simulink model "mech_ballistic_kin_fric"  (Simulink 6.0)
settings: Solver=ode45  StartTime=0.0  StopTime=inf  RelTol=1e-3
values from neighbouring files (symbols this model uses):
  m = 161    [mech_transmission_data.mat]
  N = 270    [mech_transmission_data.mat]
libraries: mblibv1 x10, simulink x1
settings Model: Creator=dkennedy  LastModifiedBy=batserve  ExtModeAutoUpdateStatusClock=off
settings DataIOCC: SignalLoggingName=sigsOut
settings DebuggingCC: CheckExecutionContextPreStartOutputMsg=on  CheckExecutionContextRuntimeOutputMsg=on  SolverPrmCheckMsg=none
settings HardwareCC: TargetUnknown=on

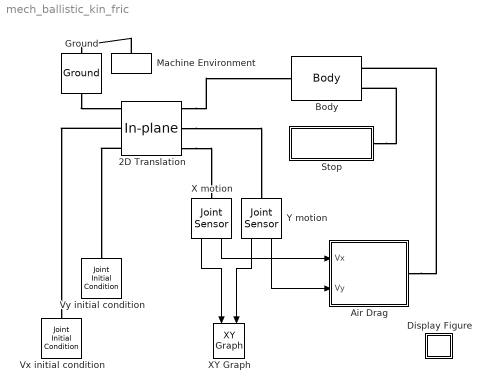
== system mech_ballistic_kin_fric ==
  2D Translation : mblibv1/Joints/In-plane  PhysicalDomain=mechanical  SubClassName=Unknown  LeftPortType=blob  RightPortType=blob  LConnTagsString=__newl0|SA1|SA2  RConnTagsString=__newr0|SA1|SA2  NumSAPorts=4  CutJoint=off  MarkAsCut=off  Primitives=prismatic_prismatic  PrimitiveProps=P1$WORLD$[1 0 0]$prismatic#P2$WORLD$[0 1 0]$prismatic  DialogClass=JointBlock
  Air Drag : Subsystem  mask(Air friction model){Cd=0}
      mask prompts: Cd "Drag Coefficient"
      mask help: Models aerodynamic drag. The drag coefficient Cd is a mask block parameter. Cd = 0 corresponds to zero drag. Cd = 2 corresponds to a sphere.
      mask init:
      | 0;
      mask Help: Enter aerodynamic drag coefficient Cd.  The block generates a three-vector of air friction as a function of 2D input velocity.
  Body : mblibv1/Bodies/Body  PhysicalDomain=mechanical  SubClassName=Unknown  LeftPortType=workingframe  RightPortType=workingframe  LConnTagsString=CS1  RConnTagsString=CS2|CG  DialogClass=MechanicalBodyBlock  Mass=100  MassUnits=kg  InertiaUnits=kg*m^2  Inertia=eye(3)*10  Shape=Cylinder  ShapeDims=[1 1]  ShapeUnits=m  ShapeUse=false  Density=1  DensityUnits=kg/m^3  DensityUse=false  CG=Right$CG$[0 0 0]$WORLD$WORLD$m$[0 0 0]$Euler X-Y-Z$deg$WORLD$true  WorkingFrames=Left$CS1$[0 0 0]$WORLD$CG$m$[0 0 0]$Euler X-Y-Z$deg$WORLD$true#Right$CS2$[0 0 0]$WORLD$CG$m$[0 0 0]$Euler X-Y-Z$deg$WORLD$true
  Display Figure : Subsystem  Tag=Help  Description="Help callback for ballistic kinetic friction model: mech_ballistic_kin_fric.  Opens Help browser to Type 19 marker at documentation for this tutorial model."
      settings: OpenFcn=pmhelpview([docroot '/toolbox/physmod/mech/mech.map'], 'mech_ballistic_kin_fric_help');
      mask Type: Help callback
      mask Display: image(imread('info.bmp'))
  Ground : mblibv1/Bodies/Ground  Orientation=down  Opaque=on  LeftPortType=env  RightPortType=workingframe  PhysicalDomain=Mechanical  DialogClass=GroundBlock  CoordPosition=[0 0 0]  CoordPositionUnits=m  StateVectorMgrId=-1  MachineId=[0 0]  ShowEnvPort=on
  Machine Environment : mblibv1/Bodies/Machine Environment  Tag=Factory ground  Orientation=up  DialogController=MECH.DialogSource  Opaque=on  PortType=env  PhysicalDomain=Mechanical  DialogTemplateClass=MECH.MachineEnvironment  SyncWhenCopied=off  Gravity=[0 -9.81 0]  GravityUnits=m/s^2  GravityAsSignal=off  Dimensionality=3D Only  AnalysisType=Forward dynamics  LinearAssemblyTolerance=1e-3  LinearAssemblyToleranceUnits=m  AngularAssemblyTolerance=1e-3  AngularAssemblyToleranceUnits=rad  ConstraintSolverType=Stabilizing  ConstraintRelTolerance=1e-4  ConstraintAbsTolerance=1e-4  UseRobustSingularityHandling=off  StatePerturbationType=Fixed  PerturbationSize=1e-5  VisualizeMachine=on
  Stop : Subsystem  Orientation=left
  Vx initial condition : mblibv1/Sensors &  Actuators/Joint Initial Condition  Orientation=up  Opaque=on  PhysicalDomain=Mechanical  DialogClass=InitialConditionBlock  Primitive=P1  CoordPosition=0.0  Velocity=98.0  AngleUnits=deg  ArcVelocityUnits=deg/s  CoordPositionUnits=m  VelocityUnits=m/s  InitialConditions=P1$true$0.0$m$deg$98.0$m/s$deg/s#P2$false$0$m$rad$0$m/s$rad/s#P3$false$0$m$rad$0$m/s$rad/s#R1$false$0$m$rad$0$m/s$rad/s#R2$false$0$m$rad$0$m/s$rad/s#R3$false$0$m$rad$0$m/s$rad/s#S$false$0$m$rad$0$m/s$rad/s
  Vy initial condition : mblibv1/Sensors &  Actuators/Joint Initial Condition  Orientation=up  Opaque=on  PhysicalDomain=Mechanical  DialogClass=InitialConditionBlock  Primitive=P2  CoordPosition=0.0  Velocity=69.0  AngleUnits=deg  ArcVelocityUnits=deg/s  CoordPositionUnits=m  VelocityUnits=m/s  InitialConditions=P1$false$0$m$rad$0$m/s$rad/s#P2$true$0.0$m$deg$69.0$m/s$deg/s#P3$false$0$m$rad$0$m/s$rad/s#R1$false$0$m$rad$0$m/s$rad/s#R2$false$0$m$rad$0$m/s$rad/s#R3$false$0$m$rad$0$m/s$rad/s#S$false$0$m$rad$0$m/s$rad/s
  X motion : mblibv1/Sensors &  Actuators/Joint Sensor  Orientation=down  Opaque=on  PhysicalDomain=Mechanical  PortType=blob  Muxed=off  Pose=off  Angle=on  AngleUnits=deg  ArcVelocity=off  ArcVelocityUnits=deg/s  ArcAcceleration=off  ArcAccelerationUnits=deg/s^2  CoordPosition=on  CoordPositionUnits=m  Velocity=on  VelocityUnits=m/s  Acceleration=off  AccelerationUnits=m/s^2  Quaternion=on  QuaternionDT=off  QuaternionDDT=off  QuaternionUnits=off  OutputVector=[ 1 1 ]  ActiveIO=on  Width=2  DialogClass=MechanicalSensorBlock  Primitive=P1  Force=off  ForceUnits=N  Torque=off  TorqueUnits=N-m  ReferenceFrame=Absolute (INERTIAL)  ReactionSensedSide=Base  ReactionReferenceFrame=Absolute (World)  ReactionForce=off  ReactionForceUnits=N  ReactionMoment=off  ReactionMomentUnits=N-m
  XY Graph : simulink/Sinks/XY Graph  Orientation=down  xmin=0  xmax=1500  ymin=0  ymax=400  st=-1
  Y motion : mblibv1/Sensors &  Actuators/Joint Sensor  Orientation=down  Opaque=on  PhysicalDomain=Mechanical  PortType=blob  Muxed=off  Pose=off  Angle=on  AngleUnits=deg  ArcVelocity=off  ArcVelocityUnits=deg/s  ArcAcceleration=off  ArcAccelerationUnits=deg/s^2  CoordPosition=on  CoordPositionUnits=m  Velocity=on  VelocityUnits=m/s  Acceleration=off  AccelerationUnits=m/s^2  Quaternion=on  QuaternionDT=off  QuaternionDDT=off  QuaternionUnits=off  OutputVector=[ 1 1 ]  ActiveIO=on  Width=2  DialogClass=MechanicalSensorBlock  Primitive=P2  Force=off  ForceUnits=N  Torque=off  TorqueUnits=N-m  ReferenceFrame=Absolute (INERTIAL)  ReactionSensedSide=Base  ReactionReferenceFrame=Absolute (World)  ReactionForce=off  ReactionForceUnits=N  ReactionMoment=off  ReactionMomentUnits=N-m
  wires:
  X motion/2 -> Air Drag/1(Vx)
  Y motion/2 -> Air Drag/2(Vy)
  X motion/1 -> XY Graph/1
  Y motion/1 -> XY Graph/2
  connections:
  Ground/RConn1 -- 2D Translation/LConn1
  2D Translation/LConn2 -- Vx initial condition/RConn1
  2D Translation/RConn3 -- X motion/LConn1
  2D Translation/RConn2 -- Y motion/LConn1
  2D Translation/LConn3 -- Vy initial condition/RConn1
  Air Drag/RConn1 -- Body/RConn1
  2D Translation/RConn1 -- Body/LConn1
  Stop/LConn1 -- Body/RConn2
  Machine Environment/RConn1 -- Ground/LConn1

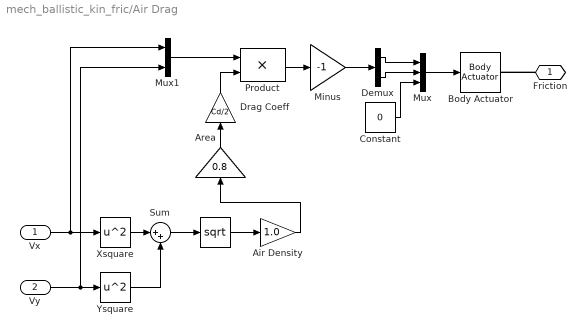
== system mech_ballistic_kin_fric/Air Drag ==
  Vx : Inport  Port=1  LatchInput=off
  Vy : Inport  Port=2  LatchInput=off
  " " : Math  Operator=sqrt  SaturateOnIntegerOverflow=on
  Air Density : Gain  Gain=1.0  SaturateOnIntegerOverflow=on
  Area : Gain  Orientation=up  Gain=0.8  SaturateOnIntegerOverflow=on
  Body Actuator : mblibv1/Sensors &  Actuators/Body Actuator  Opaque=on  PhysicalDomain=Mechanical  PortType=blob  ActuationStyle=Force  AngleUnits=deg  ArcVelocityUnits=deg/s  ArcAccelerationUnits=deg/s^2  CoordPositionUnits=m  VelocityUnits=m/s  AccelerationUnits=m/s^2  ForceUnits=N  TorqueUnits=N-m  ActiveIO=on  Width=3  DialogClass=MechanicalActuatorBlock  ReferenceFrame=Absolute (World)  Angle=off  CoordPosition=on  Force=on  Torque=off
  Constant : Constant  Value=0
  Demux : Demux  Outputs=2
  Drag Coeff : Gain  Orientation=up  Gain=Cd/2  SaturateOnIntegerOverflow=on
  Minus : Gain  Gain=-1  SaturateOnIntegerOverflow=on
  Mux : Mux  Inputs=3
  Mux1 : Mux  Inputs=2
  Product : Product  SaturateOnIntegerOverflow=on
  Sum : Sum  Inputs=|++  SaturateOnIntegerOverflow=on
  Xsquare : Math  Operator=square  SaturateOnIntegerOverflow=on
  Ysquare : Math  Operator=square  SaturateOnIntegerOverflow=on
  Friction : PMIOPort  Orientation=left  Port=1  Side=Right
  wires:
  Vx/1 -> Mux1/1, Xsquare/1
  Xsquare/1 -> Sum/1
  Ysquare/1 -> Sum/2
  Mux/1 -> Body Actuator/1
  Constant/1 -> Mux/3
  Area/1 -> Drag Coeff/1
  Mux1/1 -> Product/1
  Vy/1 -> Mux1/2, Ysquare/1
  Drag Coeff/1 -> Product/2
  Air Density/1 -> Area/1
  Sum/1 -> " "/1
  " "/1 -> Air Density/1
  Product/1 -> Minus/1
  Minus/1 -> Demux/1
  Demux/2 -> Mux/2
  Demux/1 -> Mux/1
  connections:
  Friction/RConn1 -- Body Actuator/RConn1

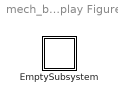
== system mech_ballistic_kin_fric/Display Figure ==
  EmptySubsystem : Subsystem

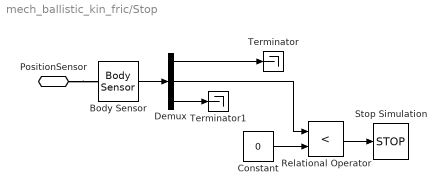
== system mech_ballistic_kin_fric/Stop ==
  Body Sensor : mblibv1/Sensors &  Actuators/Body Sensor  Opaque=on  PhysicalDomain=Mechanical  PortType=blob  Muxed=on  Pose=off  Angle=on  AngleUnits=deg  ArcVelocity=off  ArcVelocityUnits=deg/s  ArcAcceleration=off  ArcAccelerationUnits=deg/s^2  CoordPosition=on  CoordPositionUnits=m  Velocity=off  VelocityUnits=m/s  Acceleration=off  AccelerationUnits=m/s^2  Quaternion=on  QuaternionDT=off  QuaternionDDT=off  QuaternionUnits=off  OutputVector=[ 3 ]  ActiveIO=on  Width=3  DialogClass=MechanicalSensorBlock  ReferenceFrame=Absolute (World)
  Constant : Constant  Value=0
  Demux : Demux  Outputs=3
  Relational Operator : RelationalOperator  Operator=<
  Stop Simulation : Stop
  Terminator : Terminator
  Terminator1 : Terminator
  PositionSensor : PMIOPort  Port=1  Side=Left
  wires:
  Constant/1 -> Relational Operator/2
  Relational Operator/1 -> Stop Simulation/1
  Body Sensor/1 -> Demux/1
  Demux/2 -> Relational Operator/1
  Demux/1 -> Terminator/1
  Demux/3 -> Terminator1/1
  connections:
  PositionSensor/RConn1 -- Body Sensor/LConn1

== system mech_ballistic_kin_fric/Display Figure/EmptySubsystem ==
